simulink model "Ex4_5"  (R2016b)
settings: Solver=ode23s  StartTime=0.0  StopTime=1000  RelTol=1e-3
values from neighbouring files (symbols this model uses):
  alphaA = 1000/80    (= 12.5)    [ex4_3_init.m]
  g = 9.81    [ex4_3_init.m]
  Gaf = 1.273    [ex4_3_init.m]    (also in ex4_5_init.m = 0.8858)
  i_f_0 = Uf/Rf    (= 1.1)    [ex4_3_init.m]
  J2 = 10000    [ex4_3_init.m]
  Kp_i = 0.22    [ex4_3_init.m]    (also in ex4_5_init.m = 1000)
  Kp_w = 10000000    [ex4_3_init.m]    (also in ex4_5_init.m = 1000)
  m = 142.7    [ex4_3_init.m]    (also in ex4_5_init.m = 110000)
  Pnoload = 500    [ex4_3_init.m]
  r = 0.1    [ex4_3_init.m]
  Ra = 0.05    [ex4_3_init.m]    (also in ex4_5_init.m = 0.1442)
  Rf = 200    [ex4_3_init.m]    (also in ex4_5_init.m = 375)
  t_a = La/Ra    (= 0.04)    [ex4_3_init.m]
  t_f = Lf/Rf    (= 1)    [ex4_3_init.m]
  tau = 20*60    (= 1200)    [ex4_3_init.m]
  tau_u = 0.002    [ex4_3_init.m]
  Ti_i = 5.4    [ex4_3_init.m]    (also in ex4_5_init.m = 50)
  Ti_w = 0.01    [ex4_3_init.m]    (also in ex4_5_init.m = 15)
undefined symbols (not defined in the file or in its folder): sigbuilder_block
libraries: simulink x1
settings Model: Creator=Niels  LastModifiedBy=Niels

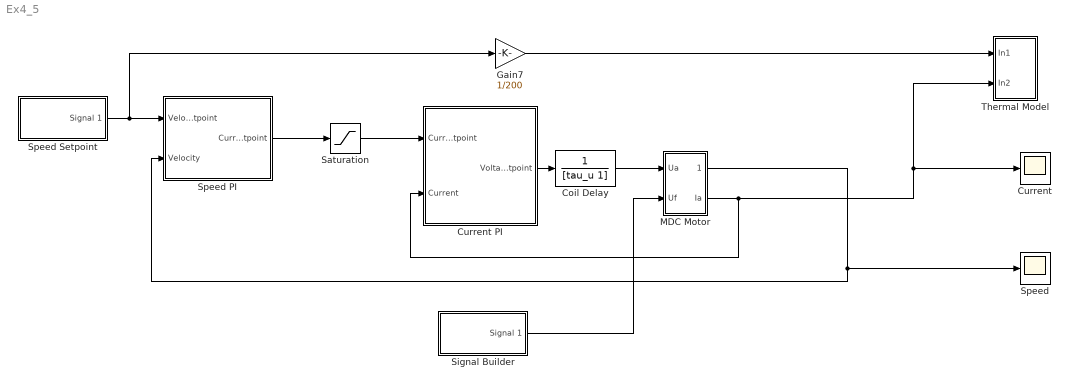
== system Ex4_5 ==
  Coil Delay : TransferFcn  Denominator=[tau_u 1]
  "Current " : Scope
  Current PI : Subsystem
  Gain7 : Gain  Gain=1/200
  MDC Motor : Subsystem
  Saturation : Saturate  UpperLimit=100  LowerLimit=-100
  Signal Builder : Subsystem  Tag=STV Subsys  LoadFcn=sigbuilder_block('load');  StartFcn=sigbuilder_block('start');  StopFcn=sigbuilder_block('stop');  ClipboardFcn=sigbuilder_block('clipboard');  mask(Sigbuilder block){tuvar=[0:10]}
      mask help: Simulink:masks:SigbuilderBlock_MD
      mask init:
      | if ~strcmp(get_param(bdroot(gcbh),'SimulationStatus'),'stopped') tuvar = sigbuilder_block('maskInit'); end
      settings: CopyFcn=sigbuilder_block('copy');  DeleteFcn=sigbuilder_block('delete');  ModelCloseFcn=sigbuilder_block('modelClose');  PreSaveFcn=sigbuilder_block('preSave');  PauseFcn=sigbuilder_block('pause');  ContinueFcn=sigbuilder_block('continue');  NameChangeFcn=sigbuilder_block('namechange');  OpenFcn=sigbuilder_block('open',[437.6 199.2 550.4 400 ]);  CloseFcn=sigbuilder_block('close');
      mask Display: plot(0, 0, 100, 100,[2, 2, 32, 32, 2], [68, 8, 8, 68, 68],[32, 2], [38, 38], [32, 19, 2],[53, 60, 44], [32, 17, 17, 2],[16, 16, 31, 31]);txt = getActiveGroup(gcbh);text(2, 100, txt,'verticalAlignment', 'top');
  Speed : Scope
  Speed PI : Subsystem
  Speed Setpoint : Subsystem  Tag=STV Subsys  LoadFcn=sigbuilder_block('load');  StartFcn=sigbuilder_block('start');  StopFcn=sigbuilder_block('stop');  ClipboardFcn=sigbuilder_block('clipboard');  mask(Sigbuilder block){tuvar=[0:10]}
      mask help: Simulink:masks:SigbuilderBlock_MD
      mask init:
      | if ~strcmp(get_param(bdroot(gcbh),'SimulationStatus'),'stopped') tuvar = sigbuilder_block('maskInit'); end
      settings: CopyFcn=sigbuilder_block('copy');  DeleteFcn=sigbuilder_block('delete');  ModelCloseFcn=sigbuilder_block('modelClose');  PreSaveFcn=sigbuilder_block('preSave');  PauseFcn=sigbuilder_block('pause');  ContinueFcn=sigbuilder_block('continue');  NameChangeFcn=sigbuilder_block('namechange');  OpenFcn=sigbuilder_block('open',[6 30 1428 681.75 ]);  CloseFcn=sigbuilder_block('close');
      mask Display: plot(0, 0, 100, 100,[2, 2, 32, 32, 2], [68, 8, 8, 68, 68],[32, 2], [38, 38], [32, 19, 2],[53, 60, 44], [32, 17, 17, 2],[16, 16, 31, 31]);txt = getActiveGroup(gcbh);text(2, 100, txt,'verticalAlignment', 'top');
  Thermal Model : Subsystem
  wires:
  Speed Setpoint/1(Signal 1) -> Gain7/1, Speed PI/1(Velocity Setpoint)
  Current PI/1(Voltage Setpoint) -> Coil Delay/1
  Speed PI/1(Current Setpoint) -> Saturation/1
  Saturation/1 -> Current PI/1(Current Setpoint)
  Gain7/1 -> Thermal Model/1(In1)
  MDC Motor/2(Ia) -> "Current "/1, Thermal Model/2(In2), Current PI/2(Current)
  Coil Delay/1 -> MDC Motor/1(Ua)
  MDC Motor/1(Wm) -> Speed/1, Speed PI/2(Velocity)
  Signal Builder/1(Signal 1) -> MDC Motor/2(Uf)

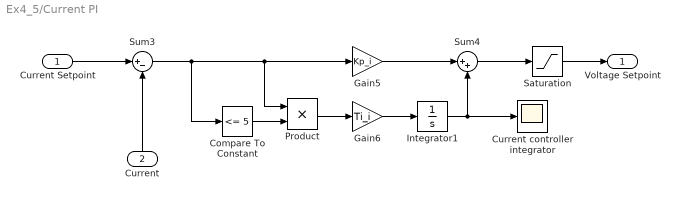
== system Ex4_5/Current PI ==
  Current Setpoint : Inport
  Current : Inport  Port=2
  Compare To Constant : simulink/Logic and Bit Operations/Compare To Constant  relop=<=  const=5  OutDataTypeStr=boolean
  Current controller integrator : Scope
  Gain5 : Gain  Gain=Kp_i
  Gain6 : Gain  Gain=Ti_i
  Integrator1 : Integrator
  Product : Product
  Saturation : Saturate  UpperLimit=220  LowerLimit=-220
  Sum3 : Sum  Inputs=|+-
  Sum4 : Sum  Inputs=|++
  Voltage Setpoint : Outport
  wires:
  Sum3/1 -> Compare To Constant/1, Product/1, Gain5/1
  Current Setpoint/1 -> Sum3/1
  Sum4/1 -> Saturation/1
  Current/1 -> Sum3/2
  Integrator1/1 -> Current controller integrator/1, Sum4/2
  Gain6/1 -> Integrator1/1
  Gain5/1 -> Sum4/1
  Saturation/1 -> Voltage Setpoint/1
  Product/1 -> Gain6/1
  Compare To Constant/1 -> Product/2

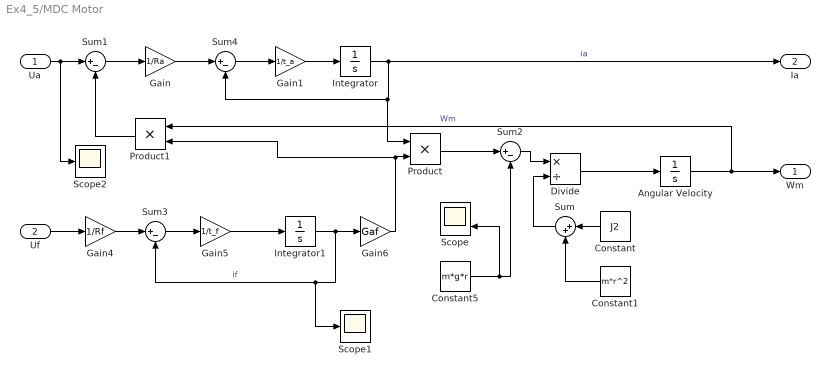
== system Ex4_5/MDC Motor ==
  Ua : Inport
  Uf : Inport  Port=2
  Angular Velocity : Integrator
  Constant : Constant  Value=J2
  Constant1 : Constant  Value=m*r^2
  Constant5 : Constant  Value=m*g*r
  Divide : Product  Inputs=*/
  Gain : Gain  Gain=1/Ra
  Gain1 : Gain  Gain=1/t_a
  Gain4 : Gain  Gain=1/Rf
  Gain5 : Gain  Gain=1/t_f
  Gain6 : Gain  Gain=Gaf
  Integrator : Integrator
  Integrator1 : Integrator  InitialCondition=i_f_0
  Product : Product
  Product1 : Product
  Scope : Scope  NumInputPorts=2
  Scope1 : Scope
  Scope2 : Scope
  Sum : Sum  Inputs=|++
  Sum{1..4} (4 alike) : Sum  Inputs=|+-
  Wm : Outport
  Ia : Outport  Port=2
  wires:
  Constant/1 -> Sum/1
  Sum/1 -> Divide/2
  Constant1/1 -> Sum/2
  Angular Velocity/1 -> Product1/1, Wm/1  "Wm"
  Sum2/1 -> Divide/1
  Constant5/1 -> Scope/2, Sum2/2
  Divide/1 -> Angular Velocity/1
  Uf/1 -> Gain4/1
  Gain4/1 -> Sum3/1
  Sum3/1 -> Gain5/1
  Gain5/1 -> Integrator1/1
  Integrator1/1 -> Gain6/1, Scope1/1, Sum3/2  "if"
  Gain6/1 -> Product1/2, Product/2
  Product/1 -> Sum2/1
  Ua/1 -> Scope2/1, Sum1/1
  Sum1/1 -> Gain/1
  Gain/1 -> Sum4/1
  Sum4/1 -> Gain1/1
  Gain1/1 -> Integrator/1
  Integrator/1 -> Ia/1, Product/1, Sum4/2  "ia"
  Product1/1 -> Sum1/2

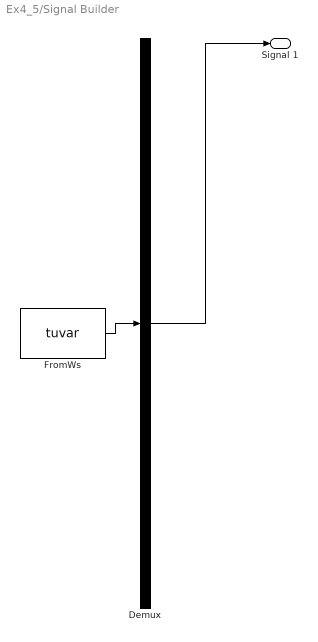
== system Ex4_5/Signal Builder ==
  Demux : Demux  Tag=STV Demux  Outputs=1
  FromWs : FromWorkspace  Tag=STV FromWs  VariableName=tuvar  SampleTime=0
      SigBuilderData=|
      | common.afterFinalStr = 'Extrapolate'
      | common.sampleTime = 0
      | dataSet.timeRange = [0 5000]
      | dataSet.name = 'Group 1'
      | sbobj.Groups.Name = 'Group 1'
      | sbobj.Groups.Signals.Name = 'Signal 1'
      | sbobj.Groups.Signals.XData = [0 5000]
      | sbobj.Groups.Signals.YData = [220 220]
      | sbobj.Groups.TimeRange = [0 5000]
  Signal 1 : Outport  Tag=STV Outport
  wires:
  Demux/1 -> Signal 1/1
  FromWs/1 -> Demux/1

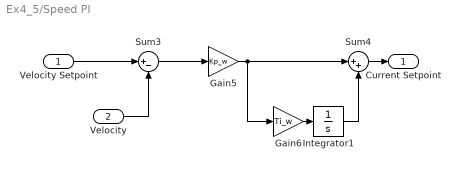
== system Ex4_5/Speed PI ==
  Velocity Setpoint : Inport
  Velocity : Inport  Port=2
  Gain5 : Gain  Gain=Kp_w
  Gain6 : Gain  Gain=Ti_w
  Integrator1 : Integrator
  Sum3 : Sum  Inputs=|+-
  Sum4 : Sum  Inputs=|++
  Current Setpoint : Outport
  wires:
  Gain6/1 -> Integrator1/1
  Sum4/1 -> Current Setpoint/1
  Velocity/1 -> Sum3/2
  Sum3/1 -> Gain5/1
  Velocity Setpoint/1 -> Sum3/1
  Gain5/1 -> Sum4/1, Gain6/1
  Integrator1/1 -> Sum4/2

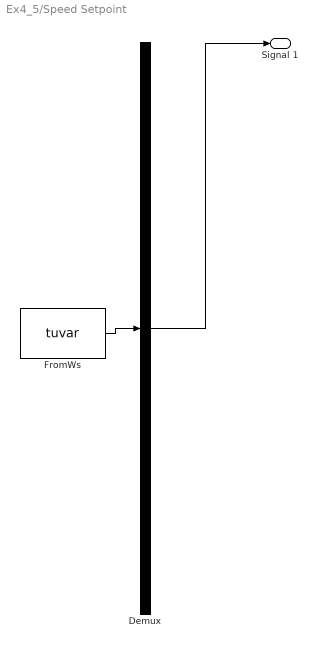
== system Ex4_5/Speed Setpoint ==
  Demux : Demux  Tag=STV Demux  Outputs=1
  FromWs : FromWorkspace  Tag=STV FromWs  VariableName=tuvar  SampleTime=0
      SigBuilderData=|
      | common.afterFinalStr = 'Extrapolate'
      | common.sampleTime = 0
      | dataSet.timeRange = [0 5000]
      | dataSet.name = 'Group 1'
      | sbobj.Groups.Name = 'Group 1'
      | sbobj.Groups.Signals.Name = 'Signal 1'
      | sbobj.Groups.Signals.XData = [0 5000]
      | sbobj.Groups.Signals.YData = [0 0]
      | sbobj.Groups.TimeRange = [0 5000]
  Signal 1 : Outport  Tag=STV Outport
  wires:
  Demux/1 -> Signal 1/1
  FromWs/1 -> Demux/1

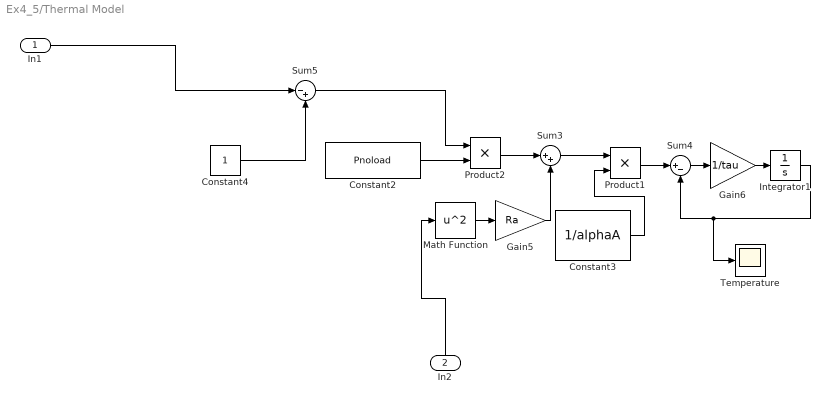
== system Ex4_5/Thermal Model ==
  In1 : Inport
  In2 : Inport  Port=2
  Constant2 : Constant  Value=Pnoload
  Constant3 : Constant  Value=1/alphaA
  Constant4 : Constant
  Gain5 : Gain  Gain=Ra
  Gain6 : Gain  Gain=1/tau
  Integrator1 : Integrator
  Math Function : Math  Operator=square  SaturateOnIntegerOverflow=on
  Product1 : Product
  Product2 : Product
  Sum3 : Sum  Inputs=|++
  Sum4 : Sum  Inputs=|+-
  Sum5 : Sum  Inputs=|-+
  Temperature : Scope
  wires:
  In2/1 -> Math Function/1
  Product2/1 -> Sum3/1
  Sum5/1 -> Product2/1
  Constant2/1 -> Product2/2
  Math Function/1 -> Gain5/1
  Product1/1 -> Sum4/1
  In1/1 -> Sum5/1
  Gain6/1 -> Integrator1/1
  Sum4/1 -> Gain6/1
  Integrator1/1 -> Temperature/1, Sum4/2
  Gain5/1 -> Sum3/2
  Constant4/1 -> Sum5/2
  Sum3/1 -> Product1/1
  Constant3/1 -> Product1/2
